simulink model "Antiwindup_PID_with_clamping"  (R2018a)
settings: Solver=FixedStepAuto  StartTime=0.0  StopTime=10.0  RelTol=1e-3
libraries: simulink x1
settings Model: Creator=CREATIVEDESK  LastModifiedBy=CREATIVEDESK

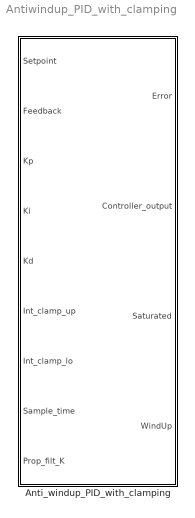
== system Antiwindup_PID_with_clamping ==
  Anti_windup_PID_with_clamping : Subsystem

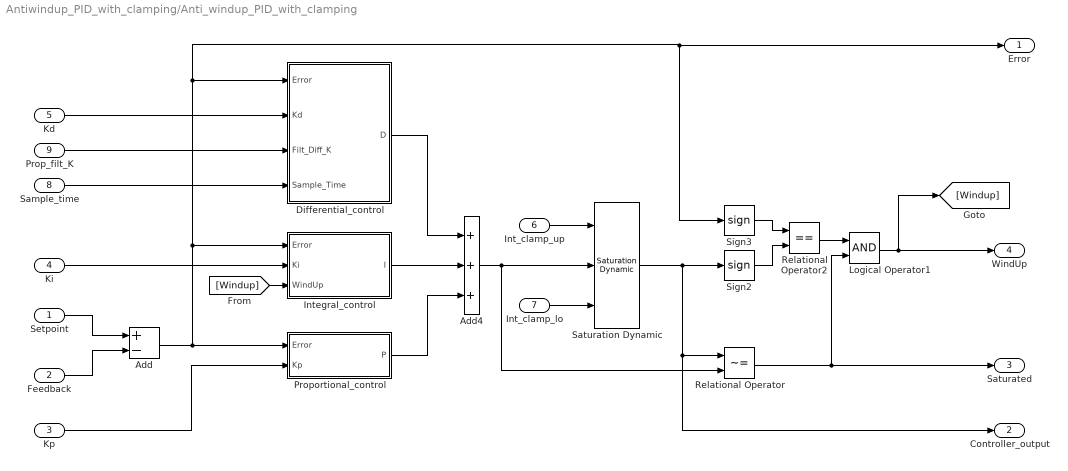
== system Antiwindup_PID_with_clamping/Anti_windup_PID_with_clamping ==
  Setpoint : Inport
  Feedback : Inport  Port=2
  Kp : Inport  Port=3
  Ki : Inport  Port=4
  Kd : Inport  Port=5
  Int_clamp_up : Inport  Port=6
  Int_clamp_lo : Inport  Port=7
  Sample_time : Inport  Port=8
  Prop_filt_K : Inport  Port=9
  Add : Sum  Inputs=+-
  Add4 : Sum  Inputs=3
  Differential_control : Subsystem
  Integral_control : Subsystem
  Logical Operator1 : Logic  AllPortsSameDT=off  OutDataTypeStr=boolean
  Proportional_control : Subsystem
  Relational Operator : RelationalOperator  Operator=~=  OutDataTypeStr=boolean  RndMeth=Simplest
  Relational Operator2 : RelationalOperator  Operator===  OutDataTypeStr=boolean  RndMeth=Simplest
  Saturation Dynamic : simulink/Discontinuities/Saturation Dynamic  OutMin=[]  OutMax=[]  OutDataTypeStr=Inherit: Same as second input  OutDataType=fixdt(1, 16)  OutScaling=2^-10  DoSatur=off
  Sign2 : Signum
  Sign3 : Signum
  Error : Outport
  Controller_output : Outport  Port=2
  Saturated : Outport  Port=3
  WindUp : Outport  Port=4
  wires:
  [Windup] -> Integral_control/3(WindUp)
  Relational Operator/1 -> Saturated/1, Logical Operator1/2
  Differential_control/1(D) -> Add4/1
  Add/1 -> Proportional_control/1(Error), Integral_control/1(Error), Differential_control/1(Error), Error/1, Sign3/1
  Ki/1 -> Integral_control/2(Ki)
  Sample_time/1 -> Differential_control/4(Sample_Time)
  Logical Operator1/1 -> WindUp/1, [Windup]
  Prop_filt_K/1 -> Differential_control/3(Filt_Diff_K)
  Add4/1 -> Relational Operator/2, Saturation Dynamic/2
  Kd/1 -> Differential_control/2(Kd)
  Sign2/1 -> Relational Operator2/2
  Saturation Dynamic/1 -> Sign2/1, Controller_output/1, Relational Operator/1
  Int_clamp_up/1 -> Saturation Dynamic/1
  Proportional_control/1(P) -> Add4/3
  Int_clamp_lo/1 -> Saturation Dynamic/3
  Kp/1 -> Proportional_control/2(Kp)
  Sign3/1 -> Relational Operator2/1
  Relational Operator2/1 -> Logical Operator1/1
  Integral_control/1(I) -> Add4/2
  Setpoint/1 -> Add/1
  Feedback/1 -> Add/2

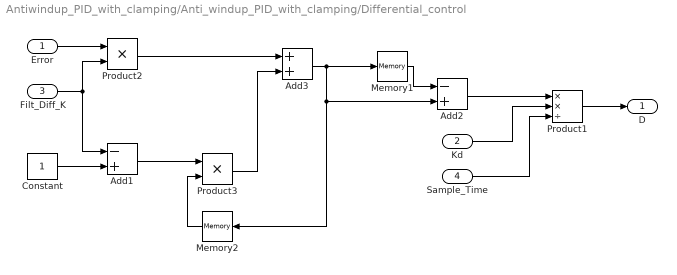
== system Antiwindup_PID_with_clamping/Anti_windup_PID_with_clamping/Differential_control ==
  Error : Inport
  Kd : Inport  Port=2
  Filt_Diff_K : Inport  Port=3
  Sample_Time : Inport  Port=4
  Add1 : Sum  Inputs=-+
  Add2 : Sum  Inputs=-+
  Add3 : Sum  Inputs=2
  Constant : Constant
  Memory1 : Memory
  Memory2 : Memory
  Product1 : Product  Inputs=**/
  Product2 : Product
  Product3 : Product
  D : Outport
  wires:
  Product1/1 -> D/1
  Kd/1 -> Product1/2
  Add2/1 -> Product1/1
  Memory1/1 -> Add2/1
  Error/1 -> Product2/1
  Filt_Diff_K/1 -> Add1/1, Product2/2
  Constant/1 -> Add1/2
  Product2/1 -> Add3/1
  Add1/1 -> Product3/1
  Product3/1 -> Add3/2
  Add3/1 -> Memory1/1, Add2/2, Memory2/1
  Memory2/1 -> Product3/2
  Sample_Time/1 -> Product1/3

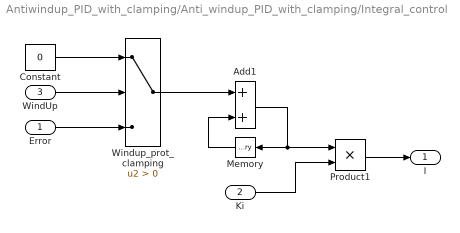
== system Antiwindup_PID_with_clamping/Anti_windup_PID_with_clamping/Integral_control ==
  Error : Inport
  Ki : Inport  Port=2
  WindUp : Inport  Port=3
  Add1 : Sum  Inputs=2
  Constant : Constant  Value=0
  Memory : Memory
  Product1 : Product
  Windup_prot_clamping : Switch  Criteria=u2 > Threshold
  I : Outport
  wires:
  Product1/1 -> I/1
  Ki/1 -> Product1/2
  Constant/1 -> Windup_prot_clamping/1
  Error/1 -> Windup_prot_clamping/3
  WindUp/1 -> Windup_prot_clamping/2
  Windup_prot_clamping/1 -> Add1/1
  Add1/1 -> Memory/1, Product1/1
  Memory/1 -> Add1/2

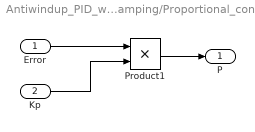
== system Antiwindup_PID_with_clamping/Anti_windup_PID_with_clamping/Proportional_control ==
  Error : Inport
  Kp : Inport  Port=2
  Product1 : Product
  P : Outport
  wires:
  Error/1 -> Product1/1
  Kp/1 -> Product1/2
  Product1/1 -> P/1
